simulink library "Pitch_System_Lib"  (Simulink 7.9)
settings: Solver=ode45  StartTime=0.0  StopTime=10.0  RelTol=1e-3
undefined symbols (not defined in the file or in its folder): WT_Params
libraries: mblibv1 x78, Pitch_Actuation_Lib x2, Pitch_System_Lib x1
(part 1 of 5)
Description:
  | Copyright 2011 MathWorks, Inc.
settings Model: Creator=smiller  LastModifiedBy=smiller

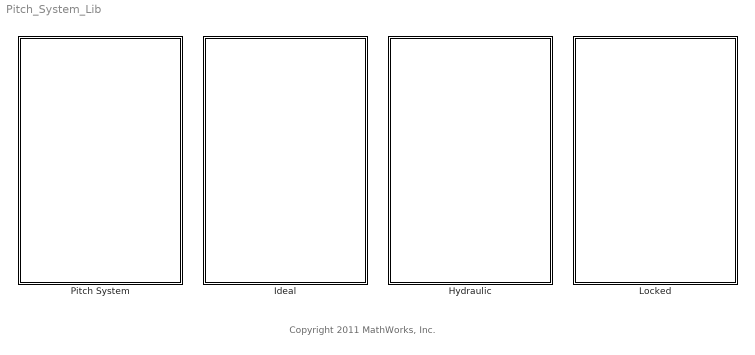
== system Pitch_System_Lib ==
  note: Copyright 2011 MathWorks, Inc.
  Hydraulic : Subsystem
      mask Display: image(imread('Pitch_Hydraulic_IMAGE.jpg'));
  Ideal : Subsystem
      mask Display: image(imread('Pitch_Ideal_IMAGE.jpg'));
  Locked : Subsystem
      mask Display: image(imread('Pitch_Locked_IMAGE.jpg'));
  Pitch System : Subsystem  BlockChoice=Hydraulic
      settings: TemplateBlock=self  MemberBlocks=Hydraulic,Ideal,Locked

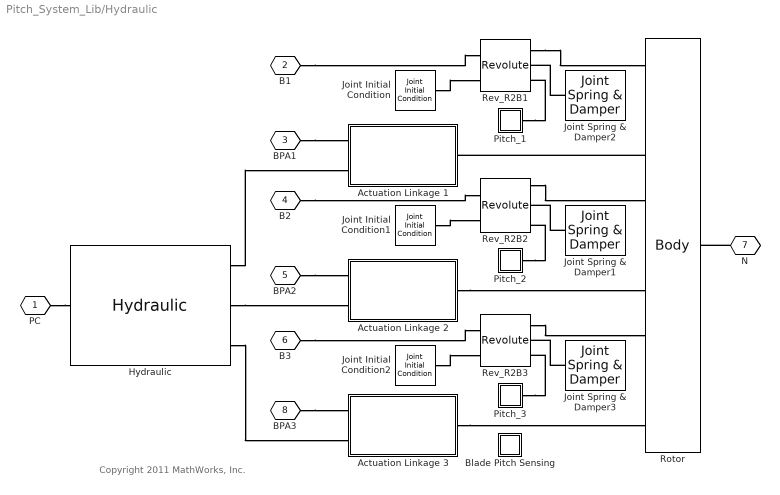
== system Pitch_System_Lib/Hydraulic ==
  note: Copyright 2011 MathWorks, Inc.
  Actuation Linkage 1 : Subsystem
      mask Display: image(imread('Pitch_Hydraulic_Linkage_IMAGE.jpg'));
  Actuation Linkage 2 : Subsystem
      mask Display: image(imread('Pitch_Hydraulic_Linkage_IMAGE.jpg'));
  Actuation Linkage 3 : Subsystem
      mask Display: image(imread('Pitch_Hydraulic_Linkage_IMAGE.jpg'));
  Blade Pitch Sensing : Subsystem
      mask Display: disp('S')
  Hydraulic : Pitch_Actuation_Lib/Hydraulic  SystemSampleTime=-1
  Joint Initial Condition : mblibv1/Sensors &  Actuators/Joint Initial Condition  SystemSampleTime=-1  UpdateFromCAD=off  LeftPortType=blob  RightPortType=blob  PhysicalDomain=mechanical  DialogClass=InitialConditionBlock  InitialConditions=P1$false$0$m$deg$0$m/s$deg/s#P2$false$0$m$deg$0$m/s$deg/s#P3$false$0$m$deg$0$m/s$deg/s#R1$true$0$m$deg$0$m/s$deg/s#R2$false$0$m$deg$0$m/s$deg/s#R3$false$0$m$deg$0$m/s$deg/s#S$false$0$m$deg$0$m/s$deg/s  P1PIC=0  P1VIC=0  P2PIC=0  P2VIC=0  P3PIC=0  P3VIC=0  R1PIC=0  R1VIC=0  R2PIC=0  R2VIC=0  R3PIC=0  R3VIC=0  SPIC=0  SVIC=0
  Joint Initial Condition1 : mblibv1/Sensors &  Actuators/Joint Initial Condition  SystemSampleTime=-1  UpdateFromCAD=off  LeftPortType=blob  RightPortType=blob  PhysicalDomain=mechanical  DialogClass=InitialConditionBlock  InitialConditions=P1$false$0$m$deg$0$m/s$deg/s#P2$false$0$m$deg$0$m/s$deg/s#P3$false$0$m$deg$0$m/s$deg/s#R1$true$0$m$deg$0$m/s$deg/s#R2$false$0$m$deg$0$m/s$deg/s#R3$false$0$m$deg$0$m/s$deg/s#S$false$0$m$deg$0$m/s$deg/s  P1PIC=0  P1VIC=0  P2PIC=0  P2VIC=0  P3PIC=0  P3VIC=0  R1PIC=0  R1VIC=0  R2PIC=0  R2VIC=0  R3PIC=0  R3VIC=0  SPIC=0  SVIC=0
  Joint Initial Condition2 : mblibv1/Sensors &  Actuators/Joint Initial Condition  SystemSampleTime=-1  UpdateFromCAD=off  LeftPortType=blob  RightPortType=blob  PhysicalDomain=mechanical  DialogClass=InitialConditionBlock  InitialConditions=P1$false$0$m$deg$0$m/s$deg/s#P2$false$0$m$deg$0$m/s$deg/s#P3$false$0$m$deg$0$m/s$deg/s#R1$true$0$m$deg$0$m/s$deg/s#R2$false$0$m$deg$0$m/s$deg/s#R3$false$0$m$deg$0$m/s$deg/s#S$false$0$m$deg$0$m/s$deg/s  P1PIC=0  P1VIC=0  P2PIC=0  P2VIC=0  P3PIC=0  P3VIC=0  R1PIC=0  R1VIC=0  R2PIC=0  R2VIC=0  R3PIC=0  R3VIC=0  SPIC=0  SVIC=0
  Joint Spring & Damper1 : mblibv1/Force  Elements/Joint Spring & Damper  SystemSampleTime=-1  UpdateFromCAD=off  DialogClass=JointSpringDamper  JFEParameters=P1$false$0$0$0$m$m/s$N$deg$deg/s$N*m#P2$false$0$0$0$m$m/s$N$deg$deg/s$N*m#P3$false$0$0$0$m$m/s$N$deg$deg/s$N*m#R1$true$0$WT_Params.Blade.damping$0$m$m/s$N$deg$deg/s$N*m#R2$false$0$0$0$m$m/s$N$deg$deg/s$N*m#R3$false$0$0$0$m$m/s$N$deg$deg/s$N*m#S$false$0$0$0$m$m/s$N$deg$deg/s$N*m
  Joint Spring & Damper2 : mblibv1/Force  Elements/Joint Spring & Damper  SystemSampleTime=-1  UpdateFromCAD=off  DialogClass=JointSpringDamper  JFEParameters=P1$false$0$0$0$m$m/s$N$deg$deg/s$N*m#P2$false$0$0$0$m$m/s$N$deg$deg/s$N*m#P3$false$0$0$0$m$m/s$N$deg$deg/s$N*m#R1$true$0$WT_Params.Blade.damping$0$m$m/s$N$deg$deg/s$N*m#R2$false$0$0$0$m$m/s$N$deg$deg/s$N*m#R3$false$0$0$0$m$m/s$N$deg$deg/s$N*m#S$false$0$0$0$m$m/s$N$deg$deg/s$N*m
  Joint Spring & Damper3 : mblibv1/Force  Elements/Joint Spring & Damper  SystemSampleTime=-1  UpdateFromCAD=off  DialogClass=JointSpringDamper  JFEParameters=P1$false$0$0$0$m$m/s$N$deg$deg/s$N*m#P2$false$0$0$0$m$m/s$N$deg$deg/s$N*m#P3$false$0$0$0$m$m/s$N$deg$deg/s$N*m#R1$true$0$WT_Params.Blade.damping$0$m$m/s$N$deg$deg/s$N*m#R2$false$0$0$0$m$m/s$N$deg$deg/s$N*m#R3$false$0$0$0$m$m/s$N$deg$deg/s$N*m#S$false$0$0$0$m$m/s$N$deg$deg/s$N*m
  Pitch_1 : Subsystem
  Pitch_2 : Subsystem
  Pitch_3 : Subsystem
  Rev_R2B1 : mblibv1/Joints/Revolute  LConnTagsString=__newl0|SA1|SA2  RConnTagsString=__newr0|SA1  UpdateFromCAD=off  NumSAPorts=3  CutJoint=off  MarkAsCut=off  Primitives=prismatic  PrimitiveProps=R1$Base$[0 -1 0]$revolute  DialogClass=JointBlock  R1Axis=[0 -1 0]
  Rev_R2B2 : mblibv1/Joints/Revolute  LConnTagsString=__newl0|SA1|SA2  RConnTagsString=__newr0|SA1  UpdateFromCAD=off  NumSAPorts=3  CutJoint=off  MarkAsCut=off  Primitives=prismatic  PrimitiveProps=R1$Base$[0 -1 0]$revolute  DialogClass=JointBlock  R1Axis=[0 -1 0]
  Rev_R2B3 : mblibv1/Joints/Revolute  LConnTagsString=__newl0|SA1|SA2  RConnTagsString=__newr0|SA1  UpdateFromCAD=off  NumSAPorts=3  CutJoint=off  MarkAsCut=off  Primitives=prismatic  PrimitiveProps=R1$Base$[0 -1 0]$revolute  DialogClass=JointBlock  R1Axis=[0 -1 0]
  Rotor : mblibv1/Bodies/Body  LConnTagsString=CS4|CS10|CS14|CS5|CS11|CS16|CS6|CS12|CS18  RConnTagsString=CG  UpdateFromCAD=off  DialogClass=MechanicalBodyBlock  Mass=WT_Params.Rotor.mass  MassUnits=kg  InertiaUnits=kg*m^2  Inertia=WT_Params.Rotor.inertia  Shape=Cylinder  ShapeDims=[1 1]  ShapeUnits=m  ShapeUse=false  Density=1  DensityUnits=kg/m^3  DensityUse=false  GraphicsMode=MACHINE_DEFAULT  BodyColorSelMode=COLORPALETTE  BodyColor=[1 1 1]  AttachedToCS=CG  CG=Right$CG$[0 0 0]$Adjoining$Adjoining$m$[0 0 0]$Euler X-Y-Z$deg$Adjoining$true$none  WorkingFrames=Right$CS19$[-WT_Params.Rotor.Geometry.length 0 0]$CG$CG$m$[0 0 0]$Euler X-Y-Z$deg$Adjoining$false$none#Left$CS1$[0 0 0]$CG$CG$m$[0 0 0]$Euler X-Y-Z$deg$CG$false$none#Left$CS4$[0 WT_Params.Rotor.radius 0]$CS1$CS1$m$[0 0 0]$Euler X-Y-Z$deg$CS1$true$none#Left$CS7$[0 0 0]$CG$CG$m$[60 0 0]$Euler X-Y-Z$deg$CG$false$none#Left$CS10$[0 WT_Params.Rotor.radius 0]$CS7$CS7$m$[0 0 0]$Euler X-Y-Z$deg$CS7$true$none#Left$CS13$[-WT_Params.Rotor.Pitch_Actuator_Offset.x 0 WT_Params.Rotor.Pitch_Actuator_Offset.z]$CG$CG$m$[WT_Params.Rotor.Pitch_Actuator_Offset.angle 0 0]$Euler X-Y-Z$deg$CG$false$none#Left$CS14$[0 WT_Params.Rotor.Pitch_Actuator_Offset.y 0]$CS13$CS13$m$[0 0 0]$Euler X-Y-Z$deg$CS13$true$none#Left$CS2$[0 0 0]$CG$CG$m$[120 0 0]$Euler X-Y-Z$deg$CG$false$none#Left$CS5$[0 WT_Params.Rotor.radius 0]$CS2$CS2$m$[0 0 0]$Euler X-Y-Z$deg$CS2$true$none#Left$CS8$[0 0 0]$CG$CG$m$[180 0 0]$Euler X-Y-Z$deg$CG$false$none#Left$CS11$[0 WT_Params.Rotor.radius 0]$CS8$CS8$m$[0 0 0]$Euler X-Y-Z$deg$CS8$true$none#Left$CS15$[-WT_Params.Rotor.Pitch_Actuator_Offset.x 0 0]$CG$CG$m$[WT_Params.Rotor.Pitch_Actuator_Offset.angle+120 0 0]$Euler X-Y-Z$deg$CG$false$none#Left$CS16$[0 WT_Params.Rotor.Pitch_Actuator_Offset.y WT_Params.Rotor.Pitch_Actuator_Offset.z]$CS15$CS15$m$[0 0 0]$Euler X-Y-Z$deg$CS15$true$none#Left$CS3$[0 0 0]$CG$CG$m$[240 0 0]$Euler X-Y-Z$deg$CG$false$none#Left$CS6$[0 WT_Params.Rotor.radius 0]$CS3$CS3$m$[0 0 0]$Euler X-Y-Z$deg$CS3$true$none#Left$CS9$[0 0 0]$CG$CG$m$[300 0 0]$Euler X-Y-Z$deg$CG$false$none#Left$CS12$[0 WT_Params.Rotor.radius 0]$CS9$CS9$m$[0 0 0]$Euler X-Y-Z$deg$CS9$true$none#Left$CS17$[-WT_Params.Rotor.Pitch_Actuator_Offset.x 0 0]$CG$CG$m$[WT_Params.Rotor.Pitch_Actuator_Offset.angle+240 0 0]$Euler X-Y-Z$deg$CG$false$none#Left$CS18$[0 WT_Params.Rotor.Pitch_Actuator_Offset.y WT_Params.Rotor.Pitch_Actuator_Offset.z]$CS17$CS17$m$[0 0 0]$Euler X-Y-Z$deg$CS17$true$none  CGPos=[0 0 0]  CGRot=[0 0 0]  CS0Pos=[]  CS0Rot=[]  CS1Pos=[0 0 0]  CS1Rot=[0 0 0]  CS2Pos=[0 0 0]  CS2Rot=[120 0 0]  CS3Pos=[0 0 0]  CS3Rot=[240 0 0]  CS4Pos=[0 WT_Params.Rotor.radius 0]  CS4Rot=[0 0 0]  CS5Pos=[0 WT_Params.Rotor.radius 0]  CS5Rot=[0 0 0]  CS6Pos=[0 WT_Params.Rotor.radius 0]  CS6Rot=[0 0 0]  CS7Pos=[0 0 0]  CS7Rot=[60 0 0]  CS8Pos=[0 0 0]  CS8Rot=[180 0 0]  CS9Pos=[0 0 0]  CS9Rot=[300 0 0]  CS10Pos=[0 WT_Params.Rotor.radius 0]  CS10Rot=[0 0 0]  CS11Pos=[0 WT_Params.Rotor.radius 0]  CS11Rot=[0 0 0]  CS12Pos=[0 WT_Params.Rotor.radius 0]  CS12Rot=[0 0 0]  CS13Pos=[-WT_Params.Rotor.Pitch_Actuator_Offset.x 0 WT_Params.Rotor.Pitch_Actuator_Offset.z]  CS13Rot=[WT_Params.Rotor.Pitch_Actuator_Offset.angle 0 0]  CS14Pos=[0 WT_Params.Rotor.Pitch_Actuator_Offset.y 0]  CS14Rot=[0 0 0]  CS15Pos=[-WT_Params.Rotor.Pitch_Actuator_Offset.x 0 0]  CS15Rot=[WT_Params.Rotor.Pitch_Actuator_Offset.angle+120 0 0]  CS16Pos=[0 WT_Params.Rotor.Pitch_Actuator_Offset.y WT_Params.Rotor.Pitch_Actuator_Offset.z]  CS16Rot=[0 0 0]  CS17Pos=[-WT_Params.Rotor.Pitch_Actuator_Offset.x 0 0]  CS17Rot=[WT_Params.Rotor.Pitch_Actuator_Offset.angle+240 0 0]  CS18Pos=[0 WT_Params.Rotor.Pitch_Actuator_Offset.y WT_Params.Rotor.Pitch_Actuator_Offset.z]  CS18Rot=[0 0 0]  CS19Pos=[-WT_Params.Rotor.Geometry.length 0 0]  CS19Rot=[0 0 0]  CS20Pos=[]  CS20Rot=[]
  PC : PMIOPort  Tag=PMCPort  Port=1  Side=Left
  B1 : PMIOPort  Tag=PMCPort  Port=2  Side=Left
  BPA1 : PMIOPort  Tag=PMCPort  Port=3  Side=Left
  B2 : PMIOPort  Tag=PMCPort  Port=4  Side=Left
  BPA2 : PMIOPort  Tag=PMCPort  Port=5  Side=Left
  B3 : PMIOPort  Tag=PMCPort  Port=6  Side=Left
  N : PMIOPort  Tag=PMCPort  Port=7  Side=Right
  BPA3 : PMIOPort  Tag=PMCPort  Port=8  Side=Left
  connections:
  Pitch_1/LConn1 -- Rev_R2B1/LConn3
  B3/RConn1 -- Rev_R2B3/RConn1
  B2/RConn1 -- Rev_R2B2/RConn1
  B1/RConn1 -- Rev_R2B1/RConn1
  Rev_R2B1/LConn1 -- Rotor/LConn1
  Rev_R2B2/LConn1 -- Rotor/LConn4
  Rev_R2B3/LConn1 -- Rotor/LConn7
  Rotor/LConn3 -- Actuation Linkage 1/RConn1
  Hydraulic/RConn1 -- Actuation Linkage 1/LConn2
  BPA2/RConn1 -- Actuation Linkage 2/LConn1
  Actuation Linkage 3/RConn1 -- Rotor/LConn9
  BPA3/RConn1 -- Actuation Linkage 3/LConn1
  Actuation Linkage 2/RConn1 -- Rotor/LConn6
  BPA1/RConn1 -- Actuation Linkage 1/LConn1
  Hydraulic/RConn3 -- Actuation Linkage 3/LConn2
  PC/RConn1 -- Hydraulic/LConn1
  Hydraulic/RConn2 -- Actuation Linkage 2/LConn2
  Joint Spring & Damper1/LConn1 -- Rev_R2B2/LConn2
  Joint Spring & Damper3/LConn1 -- Rev_R2B3/LConn2
  Joint Spring & Damper2/LConn1 -- Rev_R2B1/LConn2
  Joint Initial Condition/RConn1 -- Rev_R2B1/RConn2
  Joint Initial Condition1/RConn1 -- Rev_R2B2/RConn2
  Joint Initial Condition2/RConn1 -- Rev_R2B3/RConn2
  Pitch_2/LConn1 -- Rev_R2B2/LConn3
  Pitch_3/LConn1 -- Rev_R2B3/LConn3
  N/RConn1 -- Rotor/RConn1

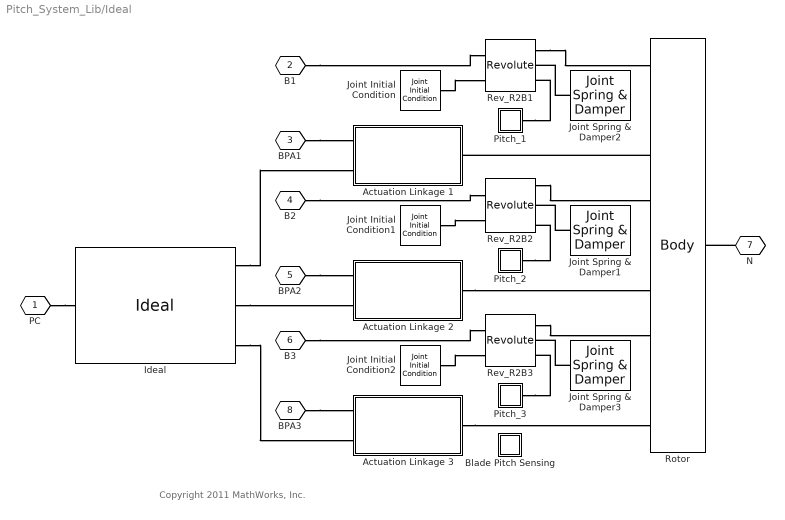
== system Pitch_System_Lib/Ideal ==
  note: Copyright 2011 MathWorks, Inc.
  Actuation Linkage 1 : Subsystem
      mask Display: image(imread('Pitch_Ideal_Linkage_IMAGE.jpg'));
  Actuation Linkage 2 : Subsystem
      mask Display: image(imread('Pitch_Ideal_Linkage_IMAGE.jpg'));
  Actuation Linkage 3 : Subsystem
      mask Display: image(imread('Pitch_Ideal_Linkage_IMAGE.jpg'));
  Blade Pitch Sensing : Subsystem
      mask Display: disp('S')
  Ideal : Pitch_Actuation_Lib/Ideal  SystemSampleTime=-1
  Joint Initial Condition : mblibv1/Sensors &  Actuators/Joint Initial Condition  SystemSampleTime=-1  UpdateFromCAD=off  LeftPortType=blob  RightPortType=blob  PhysicalDomain=mechanical  DialogClass=InitialConditionBlock  InitialConditions=P1$false$0$m$deg$0$m/s$deg/s#P2$false$0$m$deg$0$m/s$deg/s#P3$false$0$m$deg$0$m/s$deg/s#R1$true$0$m$deg$0$m/s$deg/s#R2$false$0$m$deg$0$m/s$deg/s#R3$false$0$m$deg$0$m/s$deg/s#S$false$0$m$deg$0$m/s$deg/s  P1PIC=0  P1VIC=0  P2PIC=0  P2VIC=0  P3PIC=0  P3VIC=0  R1PIC=0  R1VIC=0  R2PIC=0  R2VIC=0  R3PIC=0  R3VIC=0  SPIC=0  SVIC=0
  Joint Initial Condition1 : mblibv1/Sensors &  Actuators/Joint Initial Condition  SystemSampleTime=-1  UpdateFromCAD=off  LeftPortType=blob  RightPortType=blob  PhysicalDomain=mechanical  DialogClass=InitialConditionBlock  InitialConditions=P1$false$0$m$deg$0$m/s$deg/s#P2$false$0$m$deg$0$m/s$deg/s#P3$false$0$m$deg$0$m/s$deg/s#R1$true$0$m$deg$0$m/s$deg/s#R2$false$0$m$deg$0$m/s$deg/s#R3$false$0$m$deg$0$m/s$deg/s#S$false$0$m$deg$0$m/s$deg/s  P1PIC=0  P1VIC=0  P2PIC=0  P2VIC=0  P3PIC=0  P3VIC=0  R1PIC=0  R1VIC=0  R2PIC=0  R2VIC=0  R3PIC=0  R3VIC=0  SPIC=0  SVIC=0
  Joint Initial Condition2 : mblibv1/Sensors &  Actuators/Joint Initial Condition  SystemSampleTime=-1  UpdateFromCAD=off  LeftPortType=blob  RightPortType=blob  PhysicalDomain=mechanical  DialogClass=InitialConditionBlock  InitialConditions=P1$false$0$m$deg$0$m/s$deg/s#P2$false$0$m$deg$0$m/s$deg/s#P3$false$0$m$deg$0$m/s$deg/s#R1$true$0$m$deg$0$m/s$deg/s#R2$false$0$m$deg$0$m/s$deg/s#R3$false$0$m$deg$0$m/s$deg/s#S$false$0$m$deg$0$m/s$deg/s  P1PIC=0  P1VIC=0  P2PIC=0  P2VIC=0  P3PIC=0  P3VIC=0  R1PIC=0  R1VIC=0  R2PIC=0  R2VIC=0  R3PIC=0  R3VIC=0  SPIC=0  SVIC=0
  Joint Spring & Damper1 : mblibv1/Force  Elements/Joint Spring & Damper  SystemSampleTime=-1  UpdateFromCAD=off  DialogClass=JointSpringDamper  JFEParameters=P1$false$0$0$0$m$m/s$N$deg$deg/s$N*m#P2$false$0$0$0$m$m/s$N$deg$deg/s$N*m#P3$false$0$0$0$m$m/s$N$deg$deg/s$N*m#R1$true$0$WT_Params.Blade.damping$0$m$m/s$N$deg$deg/s$N*m#R2$false$0$0$0$m$m/s$N$deg$deg/s$N*m#R3$false$0$0$0$m$m/s$N$deg$deg/s$N*m#S$false$0$0$0$m$m/s$N$deg$deg/s$N*m
  Joint Spring & Damper2 : mblibv1/Force  Elements/Joint Spring & Damper  SystemSampleTime=-1  UpdateFromCAD=off  DialogClass=JointSpringDamper  JFEParameters=P1$false$0$0$0$m$m/s$N$deg$deg/s$N*m#P2$false$0$0$0$m$m/s$N$deg$deg/s$N*m#P3$false$0$0$0$m$m/s$N$deg$deg/s$N*m#R1$true$0$WT_Params.Blade.damping$0$m$m/s$N$deg$deg/s$N*m#R2$false$0$0$0$m$m/s$N$deg$deg/s$N*m#R3$false$0$0$0$m$m/s$N$deg$deg/s$N*m#S$false$0$0$0$m$m/s$N$deg$deg/s$N*m
  Joint Spring & Damper3 : mblibv1/Force  Elements/Joint Spring & Damper  SystemSampleTime=-1  UpdateFromCAD=off  DialogClass=JointSpringDamper  JFEParameters=P1$false$0$0$0$m$m/s$N$deg$deg/s$N*m#P2$false$0$0$0$m$m/s$N$deg$deg/s$N*m#P3$false$0$0$0$m$m/s$N$deg$deg/s$N*m#R1$true$0$WT_Params.Blade.damping$0$m$m/s$N$deg$deg/s$N*m#R2$false$0$0$0$m$m/s$N$deg$deg/s$N*m#R3$false$0$0$0$m$m/s$N$deg$deg/s$N*m#S$false$0$0$0$m$m/s$N$deg$deg/s$N*m
  Pitch_1 : Subsystem
  Pitch_2 : Subsystem
  Pitch_3 : Subsystem
  Rev_R2B1 : mblibv1/Joints/Revolute  LConnTagsString=__newl0|SA1|SA2  RConnTagsString=__newr0|SA1  UpdateFromCAD=off  NumSAPorts=3  CutJoint=off  MarkAsCut=off  Primitives=prismatic  PrimitiveProps=R1$Base$[0 -1 0]$revolute  DialogClass=JointBlock  R1Axis=[0 -1 0]
  Rev_R2B2 : mblibv1/Joints/Revolute  LConnTagsString=__newl0|SA1|SA2  RConnTagsString=__newr0|SA1  UpdateFromCAD=off  NumSAPorts=3  CutJoint=off  MarkAsCut=off  Primitives=prismatic  PrimitiveProps=R1$Base$[0 -1 0]$revolute  DialogClass=JointBlock  R1Axis=[0 -1 0]
  Rev_R2B3 : mblibv1/Joints/Revolute  LConnTagsString=__newl0|SA1|SA2  RConnTagsString=__newr0|SA1  UpdateFromCAD=off  NumSAPorts=3  CutJoint=off  MarkAsCut=off  Primitives=prismatic  PrimitiveProps=R1$Base$[0 -1 0]$revolute  DialogClass=JointBlock  R1Axis=[0 -1 0]
  Rotor : mblibv1/Bodies/Body  LConnTagsString=CS4|CS10|CS14|CS5|CS11|CS16|CS6|CS12|CS18  RConnTagsString=CG  UpdateFromCAD=off  DialogClass=MechanicalBodyBlock  Mass=WT_Params.Rotor.mass  MassUnits=kg  InertiaUnits=kg*m^2  Inertia=WT_Params.Rotor.inertia  Shape=Cylinder  ShapeDims=[1 1]  ShapeUnits=m  ShapeUse=false  Density=1  DensityUnits=kg/m^3  DensityUse=false  GraphicsMode=MACHINE_DEFAULT  BodyColorSelMode=COLORPALETTE  BodyColor=[1 1 1]  AttachedToCS=CG  CG=Right$CG$[0 0 0]$Adjoining$Adjoining$m$[0 0 0]$Euler X-Y-Z$deg$Adjoining$true$none  WorkingFrames=Right$CS19$[-WT_Params.Rotor.Geometry.length 0 0]$CG$CG$m$[0 0 0]$Euler X-Y-Z$deg$Adjoining$false$none#Left$CS1$[0 0 0]$CG$CG$m$[0 0 0]$Euler X-Y-Z$deg$CG$false$none#Left$CS4$[0 WT_Params.Rotor.radius 0]$CS1$CS1$m$[0 0 0]$Euler X-Y-Z$deg$CS1$true$none#Left$CS7$[0 0 0]$CG$CG$m$[60 0 0]$Euler X-Y-Z$deg$CG$false$none#Left$CS10$[0 WT_Params.Rotor.radius 0]$CS7$CS7$m$[0 0 0]$Euler X-Y-Z$deg$CS7$true$none#Left$CS13$[-WT_Params.Rotor.Pitch_Actuator_Offset.x 0 WT_Params.Rotor.Pitch_Actuator_Offset.z]$CG$CG$m$[WT_Params.Rotor.Pitch_Actuator_Offset.angle 0 0]$Euler X-Y-Z$deg$CG$false$none#Left$CS14$[0 WT_Params.Rotor.Pitch_Actuator_Offset.y 0]$CS13$CS13$m$[0 0 0]$Euler X-Y-Z$deg$CS13$true$none#Left$CS2$[0 0 0]$CG$CG$m$[120 0 0]$Euler X-Y-Z$deg$CG$false$none#Left$CS5$[0 WT_Params.Rotor.radius 0]$CS2$CS2$m$[0 0 0]$Euler X-Y-Z$deg$CS2$true$none#Left$CS8$[0 0 0]$CG$CG$m$[180 0 0]$Euler X-Y-Z$deg$CG$false$none#Left$CS11$[0 WT_Params.Rotor.radius 0]$CS8$CS8$m$[0 0 0]$Euler X-Y-Z$deg$CS8$true$none#Left$CS15$[-WT_Params.Rotor.Pitch_Actuator_Offset.x 0 0]$CG$CG$m$[WT_Params.Rotor.Pitch_Actuator_Offset.angle+120 0 0]$Euler X-Y-Z$deg$CG$false$none#Left$CS16$[0 WT_Params.Rotor.Pitch_Actuator_Offset.y WT_Params.Rotor.Pitch_Actuator_Offset.z]$CS15$CS15$m$[0 0 0]$Euler X-Y-Z$deg$CS15$true$none#Left$CS3$[0 0 0]$CG$CG$m$[240 0 0]$Euler X-Y-Z$deg$CG$false$none#Left$CS6$[0 WT_Params.Rotor.radius 0]$CS3$CS3$m$[0 0 0]$Euler X-Y-Z$deg$CS3$true$none#Left$CS9$[0 0 0]$CG$CG$m$[300 0 0]$Euler X-Y-Z$deg$CG$false$none#Left$CS12$[0 WT_Params.Rotor.radius 0]$CS9$CS9$m$[0 0 0]$Euler X-Y-Z$deg$CS9$true$none#Left$CS17$[-WT_Params.Rotor.Pitch_Actuator_Offset.x 0 0]$CG$CG$m$[WT_Params.Rotor.Pitch_Actuator_Offset.angle+240 0 0]$Euler X-Y-Z$deg$CG$false$none#Left$CS18$[0 WT_Params.Rotor.Pitch_Actuator_Offset.y WT_Params.Rotor.Pitch_Actuator_Offset.z]$CS17$CS17$m$[0 0 0]$Euler X-Y-Z$deg$CS17$true$none  CGPos=[0 0 0]  CGRot=[0 0 0]  CS0Pos=[]  CS0Rot=[]  CS1Pos=[0 0 0]  CS1Rot=[0 0 0]  CS2Pos=[0 0 0]  CS2Rot=[120 0 0]  CS3Pos=[0 0 0]  CS3Rot=[240 0 0]  CS4Pos=[0 WT_Params.Rotor.radius 0]  CS4Rot=[0 0 0]  CS5Pos=[0 WT_Params.Rotor.radius 0]  CS5Rot=[0 0 0]  CS6Pos=[0 WT_Params.Rotor.radius 0]  CS6Rot=[0 0 0]  CS7Pos=[0 0 0]  CS7Rot=[60 0 0]  CS8Pos=[0 0 0]  CS8Rot=[180 0 0]  CS9Pos=[0 0 0]  CS9Rot=[300 0 0]  CS10Pos=[0 WT_Params.Rotor.radius 0]  CS10Rot=[0 0 0]  CS11Pos=[0 WT_Params.Rotor.radius 0]  CS11Rot=[0 0 0]  CS12Pos=[0 WT_Params.Rotor.radius 0]  CS12Rot=[0 0 0]  CS13Pos=[-WT_Params.Rotor.Pitch_Actuator_Offset.x 0 WT_Params.Rotor.Pitch_Actuator_Offset.z]  CS13Rot=[WT_Params.Rotor.Pitch_Actuator_Offset.angle 0 0]  CS14Pos=[0 WT_Params.Rotor.Pitch_Actuator_Offset.y 0]  CS14Rot=[0 0 0]  CS15Pos=[-WT_Params.Rotor.Pitch_Actuator_Offset.x 0 0]  CS15Rot=[WT_Params.Rotor.Pitch_Actuator_Offset.angle+120 0 0]  CS16Pos=[0 WT_Params.Rotor.Pitch_Actuator_Offset.y WT_Params.Rotor.Pitch_Actuator_Offset.z]  CS16Rot=[0 0 0]  CS17Pos=[-WT_Params.Rotor.Pitch_Actuator_Offset.x 0 0]  CS17Rot=[WT_Params.Rotor.Pitch_Actuator_Offset.angle+240 0 0]  CS18Pos=[0 WT_Params.Rotor.Pitch_Actuator_Offset.y WT_Params.Rotor.Pitch_Actuator_Offset.z]  CS18Rot=[0 0 0]  CS19Pos=[-WT_Params.Rotor.Geometry.length 0 0]  CS19Rot=[0 0 0]  CS20Pos=[]  CS20Rot=[]
  PC : PMIOPort  Tag=PMCPort  Port=1  Side=Left
  B1 : PMIOPort  Tag=PMCPort  Port=2  Side=Left
  BPA1 : PMIOPort  Tag=PMCPort  Port=3  Side=Left
  B2 : PMIOPort  Tag=PMCPort  Port=4  Side=Left
  BPA2 : PMIOPort  Tag=PMCPort  Port=5  Side=Left
  B3 : PMIOPort  Tag=PMCPort  Port=6  Side=Left
  N : PMIOPort  Tag=PMCPort  Port=7  Side=Right
  BPA3 : PMIOPort  Tag=PMCPort  Port=8  Side=Left
  connections:
  N/RConn1 -- Rotor/RConn1
  Pitch_3/LConn1 -- Rev_R2B3/LConn3
  Pitch_2/LConn1 -- Rev_R2B2/LConn3
  Joint Initial Condition2/RConn1 -- Rev_R2B3/RConn2
  Joint Initial Condition1/RConn1 -- Rev_R2B2/RConn2
  Joint Initial Condition/RConn1 -- Rev_R2B1/RConn2
  Joint Spring & Damper2/LConn1 -- Rev_R2B1/LConn2
  Joint Spring & Damper3/LConn1 -- Rev_R2B3/LConn2
  Joint Spring & Damper1/LConn1 -- Rev_R2B2/LConn2
  Ideal/RConn2 -- Actuation Linkage 2/LConn2
  PC/RConn1 -- Ideal/LConn1
  Ideal/RConn3 -- Actuation Linkage 3/LConn2
  BPA1/RConn1 -- Actuation Linkage 1/LConn1
  Actuation Linkage 2/RConn1 -- Rotor/LConn6
  BPA3/RConn1 -- Actuation Linkage 3/LConn1
  Actuation Linkage 3/RConn1 -- Rotor/LConn9
  BPA2/RConn1 -- Actuation Linkage 2/LConn1
  Ideal/RConn1 -- Actuation Linkage 1/LConn2
  Rotor/LConn3 -- Actuation Linkage 1/RConn1
  Rev_R2B3/LConn1 -- Rotor/LConn7
  Rev_R2B2/LConn1 -- Rotor/LConn4
  Rev_R2B1/LConn1 -- Rotor/LConn1
  B1/RConn1 -- Rev_R2B1/RConn1
  B2/RConn1 -- Rev_R2B2/RConn1
  B3/RConn1 -- Rev_R2B3/RConn1
  Pitch_1/LConn1 -- Rev_R2B1/LConn3

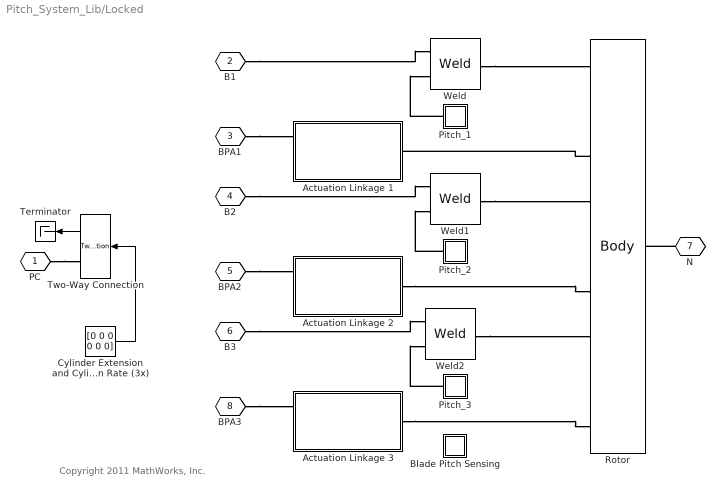
== system Pitch_System_Lib/Locked ==
  note: Copyright 2011 MathWorks, Inc.
  Actuation Linkage 1 : Subsystem
      mask Display: image(imread('Pitch_Locked_Linkage_IMAGE.jpg'))
  Actuation Linkage 2 : Subsystem
      mask Display: image(imread('Pitch_Locked_Linkage_IMAGE.jpg'))
  Actuation Linkage 3 : Subsystem
      mask Display: image(imread('Pitch_Locked_Linkage_IMAGE.jpg'))
  Blade Pitch Sensing : Subsystem
      mask Display: disp('S')
  Cylinder Extension and Cylinder Extension Rate (3x) : Constant  Value=[0 0 0 0 0 0]
  Pitch_1 : Subsystem
  Pitch_2 : Subsystem
  Pitch_3 : Subsystem
  Rotor : mblibv1/Bodies/Body  LConnTagsString=CS4|CS10|CS14|CS5|CS11|CS16|CS6|CS12|CS18  RConnTagsString=CG  UpdateFromCAD=off  DialogClass=MechanicalBodyBlock  Mass=WT_Params.Rotor.mass  MassUnits=kg  InertiaUnits=kg*m^2  Inertia=WT_Params.Rotor.inertia  Shape=Cylinder  ShapeDims=[1 1]  ShapeUnits=m  ShapeUse=false  Density=1  DensityUnits=kg/m^3  DensityUse=false  GraphicsMode=MACHINE_DEFAULT  BodyColorSelMode=COLORPALETTE  BodyColor=[1 1 1]  AttachedToCS=CG  CG=Right$CG$[0 0 0]$Adjoining$Adjoining$m$[0 0 0]$Euler X-Y-Z$deg$Adjoining$true$none  WorkingFrames=Right$CS19$[-WT_Params.Rotor.Geometry.length 0 0]$CG$CG$m$[0 0 0]$Euler X-Y-Z$deg$Adjoining$false$none#Left$CS1$[0 0 0]$CG$CG$m$[0 0 0]$Euler X-Y-Z$deg$CG$false$none#Left$CS4$[0 WT_Params.Rotor.radius 0]$CS1$CS1$m$[0 0 0]$Euler X-Y-Z$deg$CS1$true$none#Left$CS7$[0 0 0]$CG$CG$m$[60 0 0]$Euler X-Y-Z$deg$CG$false$none#Left$CS10$[0 WT_Params.Rotor.radius 0]$CS7$CS7$m$[0 0 0]$Euler X-Y-Z$deg$CS7$true$none#Left$CS13$[-WT_Params.Rotor.Pitch_Actuator_Offset.x 0 WT_Params.Rotor.Pitch_Actuator_Offset.z]$CG$CG$m$[WT_Params.Rotor.Pitch_Actuator_Offset.angle 0 0]$Euler X-Y-Z$deg$CG$false$none#Left$CS14$[0 WT_Params.Rotor.Pitch_Actuator_Offset.y 0]$CS13$CS13$m$[0 0 0]$Euler X-Y-Z$deg$CS13$true$none#Left$CS2$[0 0 0]$CG$CG$m$[120 0 0]$Euler X-Y-Z$deg$CG$false$none#Left$CS5$[0 WT_Params.Rotor.radius 0]$CS2$CS2$m$[0 0 0]$Euler X-Y-Z$deg$CS2$true$none#Left$CS8$[0 0 0]$CG$CG$m$[180 0 0]$Euler X-Y-Z$deg$CG$false$none#Left$CS11$[0 WT_Params.Rotor.radius 0]$CS8$CS8$m$[0 0 0]$Euler X-Y-Z$deg$CS8$true$none#Left$CS15$[-WT_Params.Rotor.Pitch_Actuator_Offset.x 0 0]$CG$CG$m$[WT_Params.Rotor.Pitch_Actuator_Offset.angle+120 0 0]$Euler X-Y-Z$deg$CG$false$none#Left$CS16$[0 WT_Params.Rotor.Pitch_Actuator_Offset.y WT_Params.Rotor.Pitch_Actuator_Offset.z]$CS15$CS15$m$[0 0 0]$Euler X-Y-Z$deg$CS15$true$none#Left$CS3$[0 0 0]$CG$CG$m$[240 0 0]$Euler X-Y-Z$deg$CG$false$none#Left$CS6$[0 WT_Params.Rotor.radius 0]$CS3$CS3$m$[0 0 0]$Euler X-Y-Z$deg$CS3$true$none#Left$CS9$[0 0 0]$CG$CG$m$[300 0 0]$Euler X-Y-Z$deg$CG$false$none#Left$CS12$[0 WT_Params.Rotor.radius 0]$CS9$CS9$m$[0 0 0]$Euler X-Y-Z$deg$CS9$true$none#Left$CS17$[-WT_Params.Rotor.Pitch_Actuator_Offset.x 0 0]$CG$CG$m$[WT_Params.Rotor.Pitch_Actuator_Offset.angle+240 0 0]$Euler X-Y-Z$deg$CG$false$none#Left$CS18$[0 WT_Params.Rotor.Pitch_Actuator_Offset.y WT_Params.Rotor.Pitch_Actuator_Offset.z]$CS17$CS17$m$[0 0 0]$Euler X-Y-Z$deg$CS17$true$none  CGPos=[0 0 0]  CGRot=[0 0 0]  CS0Pos=[]  CS0Rot=[]  CS1Pos=[0 0 0]  CS1Rot=[0 0 0]  CS2Pos=[0 0 0]  CS2Rot=[120 0 0]  CS3Pos=[0 0 0]  CS3Rot=[240 0 0]  CS4Pos=[0 WT_Params.Rotor.radius 0]  CS4Rot=[0 0 0]  CS5Pos=[0 WT_Params.Rotor.radius 0]  CS5Rot=[0 0 0]  CS6Pos=[0 WT_Params.Rotor.radius 0]  CS6Rot=[0 0 0]  CS7Pos=[0 0 0]  CS7Rot=[60 0 0]  CS8Pos=[0 0 0]  CS8Rot=[180 0 0]  CS9Pos=[0 0 0]  CS9Rot=[300 0 0]  CS10Pos=[0 WT_Params.Rotor.radius 0]  CS10Rot=[0 0 0]  CS11Pos=[0 WT_Params.Rotor.radius 0]  CS11Rot=[0 0 0]  CS12Pos=[0 WT_Params.Rotor.radius 0]  CS12Rot=[0 0 0]  CS13Pos=[-WT_Params.Rotor.Pitch_Actuator_Offset.x 0 WT_Params.Rotor.Pitch_Actuator_Offset.z]  CS13Rot=[WT_Params.Rotor.Pitch_Actuator_Offset.angle 0 0]  CS14Pos=[0 WT_Params.Rotor.Pitch_Actuator_Offset.y 0]  CS14Rot=[0 0 0]  CS15Pos=[-WT_Params.Rotor.Pitch_Actuator_Offset.x 0 0]  CS15Rot=[WT_Params.Rotor.Pitch_Actuator_Offset.angle+120 0 0]  CS16Pos=[0 WT_Params.Rotor.Pitch_Actuator_Offset.y WT_Params.Rotor.Pitch_Actuator_Offset.z]  CS16Rot=[0 0 0]  CS17Pos=[-WT_Params.Rotor.Pitch_Actuator_Offset.x 0 0]  CS17Rot=[WT_Params.Rotor.Pitch_Actuator_Offset.angle+240 0 0]  CS18Pos=[0 WT_Params.Rotor.Pitch_Actuator_Offset.y WT_Params.Rotor.Pitch_Actuator_Offset.z]  CS18Rot=[0 0 0]  CS19Pos=[-WT_Params.Rotor.Geometry.length 0 0]  CS19Rot=[0 0 0]  CS20Pos=[]  CS20Rot=[]
  Terminator : Terminator
  Two-Way Connection : TwoWayConnection
  Weld : mblibv1/Joints/Weld  LConnTagsString=__newl0|SA1  RConnTagsString=__newr0  UpdateFromCAD=off  NumSAPorts=1  CutJoint=off  MarkAsCut=off  Primitives=weld  PrimitiveProps=W$World$[0 0 0]$weld  DialogClass=JointBlock  WAxis=[0 0 0]
  Weld1 : mblibv1/Joints/Weld  LConnTagsString=__newl0|SA1  RConnTagsString=__newr0  UpdateFromCAD=off  NumSAPorts=1  CutJoint=off  MarkAsCut=off  Primitives=weld  PrimitiveProps=W$World$[0 0 0]$weld  DialogClass=JointBlock  WAxis=[0 0 0]
  Weld2 : mblibv1/Joints/Weld  LConnTagsString=__newl0|SA1  RConnTagsString=__newr0  UpdateFromCAD=off  NumSAPorts=1  CutJoint=off  MarkAsCut=off  Primitives=weld  PrimitiveProps=W$World$[0 0 0]$weld  DialogClass=JointBlock  WAxis=[0 0 0]
  PC : PMIOPort  Tag=PMCPort  Port=1  Side=Left
  B1 : PMIOPort  Tag=PMCPort  Port=2  Side=Left
  BPA1 : PMIOPort  Tag=PMCPort  Port=3  Side=Left
  B2 : PMIOPort  Tag=PMCPort  Port=4  Side=Left
  BPA2 : PMIOPort  Tag=PMCPort  Port=5  Side=Left
  B3 : PMIOPort  Tag=PMCPort  Port=6  Side=Left
  N : PMIOPort  Tag=PMCPort  Port=7  Side=Right
  BPA3 : PMIOPort  Tag=PMCPort  Port=8  Side=Left
  wires:
  Cylinder Extension and Cylinder Extension Rate (3x)/1 -> Two-Way Connection/1
  Two-Way Connection/1 -> Terminator/1
  connections:
  N/RConn1 -- Rotor/RConn1
  PC/RConn1 -- Two-Way Connection/RConn1
  BPA1/RConn1 -- Actuation Linkage 1/LConn1
  Actuation Linkage 2/RConn1 -- Rotor/LConn6
  BPA3/RConn1 -- Actuation Linkage 3/LConn1
  Actuation Linkage 3/RConn1 -- Rotor/LConn9
  BPA2/RConn1 -- Actuation Linkage 2/LConn1
  Rotor/LConn3 -- Actuation Linkage 1/RConn1
  Weld2/RConn1 -- Rotor/LConn7
  Weld1/RConn1 -- Rotor/LConn4
  Weld/RConn1 -- Rotor/LConn1
  B1/RConn1 -- Weld/LConn1
  B2/RConn1 -- Weld1/LConn1
  B3/RConn1 -- Weld2/LConn1
  Pitch_1/LConn1 -- Weld/LConn2
  Pitch_2/LConn1 -- Weld1/LConn2
  Pitch_3/LConn1 -- Weld2/LConn2

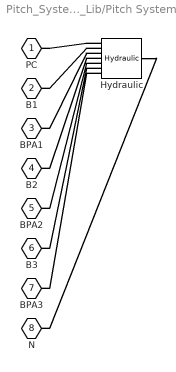
== system Pitch_System_Lib/Pitch System ==
  Hydraulic : Pitch_System_Lib/Hydraulic  SystemSampleTime=-1
  PC : PMIOPort  Port=1  Side=Left
  B1 : PMIOPort  Port=2  Side=Left
  BPA1 : PMIOPort  Port=3  Side=Left
  B2 : PMIOPort  Port=4  Side=Left
  BPA2 : PMIOPort  Port=5  Side=Left
  B3 : PMIOPort  Port=6  Side=Left
  BPA3 : PMIOPort  Port=7  Side=Left
  N : PMIOPort  Port=8  Side=Right
  connections:
  Hydraulic/LConn1 -- PC/RConn1
  Hydraulic/LConn2 -- B1/RConn1
  Hydraulic/LConn3 -- BPA1/RConn1
  Hydraulic/LConn4 -- B2/RConn1
  Hydraulic/LConn5 -- BPA2/RConn1
  Hydraulic/LConn6 -- B3/RConn1
  Hydraulic/LConn7 -- BPA3/RConn1
  Hydraulic/RConn1 -- N/RConn1

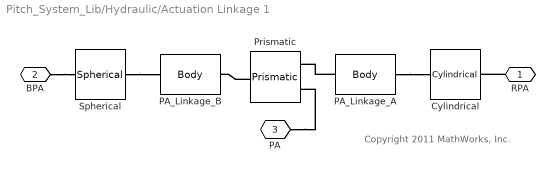
== system Pitch_System_Lib/Hydraulic/Actuation Linkage 1 ==
  note: Copyright 2011 MathWorks, Inc.
  Cylindrical : mblibv1/Joints/Cylindrical  PhysicalDomain=mechanical  SubClassName=Unknown  LeftPortType=blob  RightPortType=blob  LConnTagsString=__newl0  RConnTagsString=__newr0  UpdateFromCAD=off  NumSAPorts=0  CutJoint=off  MarkAsCut=off  Primitives=prismatic  PrimitiveProps=P1$Follower$[0 1 0]$prismatic#R1$Follower$[0 1 0]$revolute  DialogClass=JointBlock  P1Axis=[0 1 0]  R1Axis=[0 1 0]
  PA_Linkage_A : mblibv1/Bodies/Body  PhysicalDomain=mechanical  SubClassName=Unknown  LeftPortType=workingframe  RightPortType=workingframe  LConnTagsString=CS2  RConnTagsString=CS1  UpdateFromCAD=off  DialogClass=MechanicalBodyBlock  Mass=WT_Params.Pitch_Actuator.cylinder_mass  MassUnits=kg  InertiaUnits=kg*m^2  Inertia=WT_Params.Pitch_Actuator.cylinder_inertia  Shape=Cylinder  ShapeDims=[1 1]  ShapeUnits=m  ShapeUse=false  Density=1  DensityUnits=kg/m^3  DensityUse=false  GraphicsMode=MACHINE_DEFAULT  BodyColorSelMode=COLORPALETTE  BodyColor="[1     0.56863    0.011765]"  AttachedToCS=CG  CG=Left$CG$[WT_Params.Pitch_Actuator.cylinder_length/2 0 0]$CS2$CS2$m$[0 0 0]$Euler X-Y-Z$deg$CS1$false$none  WorkingFrames="Right$CS1$[WT_Params.Pitch_Actuator.cylinder_length 0 0]$CS2$CS2$m$[0 0 0]$Euler X-Y-Z$deg$Adjoining$true$none#Left$CS2$[0 0 0]$Adjoining$Adjoining$m$[0 0 0]$Euler X-Y-Z$deg$CS1$true$none#Right$CS7$[0 WT_Params.Pitch_Actuator.Geometry.outer_radius*cos(0)  WT_Params.Pitch_Actuator.Geometry.outer_radius*sin(0)]$CS1$CS1$m$[0 0 0]$Euler X-Y-Z$deg$CS1$false$none#Right$CS8$[0 WT_Params.Pitch_Actuator.Geometry.outer_radius*cos(0.2*pi)  WT_Params.Pitch_Actuator.Geometry.outer_radius*sin(0.2*pi)]$CS1$CS1$m$[0 0 0]$Euler X-Y-Z$deg$CS1$false$none#Right$CS9$[0 WT_Params.Pitch_Actuator.Geometry.outer_radius*cos(0.4*pi)  WT_Params.Pitch_Actuator.Geometry.outer_radius*sin(0.4*pi)]$CS1$CS1$m$[0 0 0]$Euler X-Y-Z$deg$CS1$false$none#Right$CS10$[0 WT_Params.Pitch_Actuator.Geometry.outer_radius*cos(0.6*pi)  WT_Params.Pitch_Actuator.Geometry.outer_radius*sin(0.6*pi)]$CS1$CS1$m$[0 0 0]$Euler X-Y-Z$deg$CS1$false$none#Right$CS11$[0 WT_Params.Pitch_Actuator.Geometry.outer_radius*cos(0.8*pi)  WT_Params.Pitch_Actuator.Geometry.outer_radius*sin(0.8*pi)]$CS1$CS1$m$[0 0 0]$Euler X-Y-Z$deg$CS1$false$none#Right$CS12$[0 WT_Params.Pitch_Actuator.Geometry.outer_radius*cos(1.0*pi)  WT_Params.Pitch_Actuator.Geometry.outer_radius*sin(1.0*pi)]$CS1$CS1$m$[0 0 0]$Euler X-Y-Z$deg$CS1$false$none#Right$CS13$[0 WT_Params.Pitch_Actuator.Geometry.outer_radius*cos(1.2*pi)  WT_Params.Pitch_Actuator.Geometry.outer_radius*sin(1.2*pi)]$CS1$CS1$m$[0 0 0]$Euler X-Y-Z$deg$CS1$false$none#Right$CS14$[0 WT_Params.Pitch_Actuator.Geometry.outer_radius*cos(1.4*pi)  WT_Params.Pitch_Actuator.Geometry.outer_radius*sin(1.4*pi)]$CS1$CS1$m$[0 0 0]$Euler X-Y-Z$deg$CS1$false$none#Right$CS15$[0 WT_Params.Pitch_Actuator.Geometry.outer_radius*cos(1.6*pi)  WT_Params.Pitch_Actuator.Geometry.outer_radius*sin(1.6*pi)]$CS1$CS1$m$[0 0 0]$Euler X-Y-Z$deg$CS1$false$none#Right$CS16$[0 WT_Params.Pitch_Actuator.Geometry.outer_radius*cos(1.8*pi)  WT_Params.Pitch_Actuator.Geometry.outer_radius*sin(1.8*pi)]$CS1$CS1$m$[0 0 0]$Euler X-Y-Z$deg$CS1$false$none#Right$CS17$[-WT_Params.Pitch_Actuator.cylinder_length WT_Params.Pitch_Actuator.Geometry.outer_radius*cos(0)  WT_Params.Pitch_Actuator.Geometry.outer_radius*sin(0)]$CS1$CS1$m$[0 0 0]$Euler X-Y-Z$deg$CS1$false$none#Right$CS18$[-WT_Params.Pitch_Actuator.cylinder_length WT_Params.Pitch_Actuator.Geometry.outer_radius*cos(0.2*pi)  WT_Params.Pitch_Actuator.Geometry.outer_radius*sin(0.2*pi)]$CS1$CS1$m$[0 0 0]$Euler X-Y-Z$deg$CS1$false$none#Right$CS19$[-WT_Params.Pitch_Actuator.cylinder_length WT_Params.Pitch_Actuator.Geometry.outer_radius*cos(0.4*pi)  WT_Params.Pitch_Actuator.Geometry.outer_radius*sin(0.4*pi)]$CS1$CS1$m$[0 0 0]$Euler X-Y-Z$deg$CS1$false$none#Right$CS20$[-WT_Params.Pitch_Actuator.cylinder_length WT_Params.Pitch_Actuator.Geometry.outer_radius*cos(0.6*pi)  WT_Params.Pitch_Actuator.Geometry.outer_radius*sin(0.6*pi)]$CS1$CS1$m$[0 0 0]$Euler X-Y-Z$deg$CS1$false$none#Right$CS21$[-WT_Params.Pitch_Actuator.cylinder_length WT_Params.Pitch_Actuator.Geometry.outer_radius*cos(0.8*pi)  WT_Params.Pitch_Actuator.Geometry.outer_radius*sin(0.8*pi)]$CS1$CS1$m$[0 0 0]$Euler X-Y-Z$deg$CS1$false$none#Right$CS22$[-WT_Params.Pitch_Actuator.cylinder_length WT_Params.Pitch_Actuator.Geometry.outer_radius*cos(1.0*pi)  WT_Params.Pitch_Actuator.Geometry.outer_radius*sin(1.0*pi)]$CS1$CS1$m$[0 0 0]$Euler X-Y-Z$deg$CS1$false$none#Right$CS23$[-WT_Params.Pitch_Actuator.cylinder_length WT_Params.Pitch_Actuator.Geometry.outer_radius*cos(1.2*pi)  WT_Params.Pitch_Actuator.Geometry.outer_radius*sin(1.2*pi)]$CS1$CS1$m$[0 0 0]$Euler X-Y-Z$deg$CS1$false$none#Right$CS24$[-WT_Params.Pitch_Actuator.cylinder_length WT_Params.Pitch_Actuator.Geometry.outer_radius*cos(1.4*pi)  WT_Params.Pitch_Actuator.Geometry.outer_radius*sin(1.4*pi)]$CS1$CS1$m$[0 0 0]$Euler X-Y-Z$deg$CS1$false$none#Right$CS25$[-WT_Params.Pitch_Actuator.cylinder_length WT_Params.Pitch_Actuator.Geometry.outer_radius*cos(1.6*pi)  WT_Params.Pitch_Actuator.Geometry.outer_radius*sin(1.6*pi)]$CS1$CS1$m$[0 0 0]$Euler X-Y-Z$deg$CS1$false$none#Right$CS26$[-WT_Params.Pitch_Actuator.cylinder_length WT_Params.Pitch_Actuator.Geometry.outer_radius*cos(1.8*pi)  WT_Params.Pitch_Actuator.Geometry.outer_radius*sin(1.8*pi)]$CS1$CS1$m$[0 0 0]$Euler X-Y-Z$deg$CS1$false$none"  CGPos=[WT_Params.Pitch_Actuator.cylinder_length/2 0 0]  CGRot=[0 0 0]  CS0Pos=[]  CS0Rot=[]  CS1Pos=[WT_Params.Pitch_Actuator.cylinder_length 0 0]  CS1Rot=[0 0 0]  CS2Pos=[0 0 0]  CS2Rot=[0 0 0]  CS3Pos=[]  CS3Rot=[]  CS4Pos=[]  CS4Rot=[]  CS5Pos=[]  CS5Rot=[]  CS6Pos=[]  CS6Rot=[]  CS7Pos="[0 WT_Params.Pitch_Actuator.Geometry.outer_radius*cos(0)  WT_Params.Pitch_Actuator.Geometry.outer_radius*sin(0)]"  CS7Rot=[0 0 0]  CS8Pos="[0 WT_Params.Pitch_Actuator.Geometry.outer_radius*cos(0.2*pi)  WT_Params.Pitch_Actuator.Geometry.outer_radius*sin(0.2*pi)]"  CS8Rot=[0 0 0]  CS9Pos="[0 WT_Params.Pitch_Actuator.Geometry.outer_radius*cos(0.4*pi)  WT_Params.Pitch_Actuator.Geometry.outer_radius*sin(0.4*pi)]"  CS9Rot=[0 0 0]  CS10Pos="[0 WT_Params.Pitch_Actuator.Geometry.outer_radius*cos(0.6*pi)  WT_Params.Pitch_Actuator.Geometry.outer_radius*sin(0.6*pi)]"  CS10Rot=[0 0 0]  CS11Pos="[0 WT_Params.Pitch_Actuator.Geometry.outer_radius*cos(0.8*pi)  WT_Params.Pitch_Actuator.Geometry.outer_radius*sin(0.8*pi)]"  CS11Rot=[0 0 0]  CS12Pos="[0 WT_Params.Pitch_Actuator.Geometry.outer_radius*cos(1.0*pi)  WT_Params.Pitch_Actuator.Geometry.outer_radius*sin(1.0*pi)]"  CS12Rot=[0 0 0]  CS13Pos="[0 WT_Params.Pitch_Actuator.Geometry.outer_radius*cos(1.2*pi)  WT_Params.Pitch_Actuator.Geometry.outer_radius*sin(1.2*pi)]"  CS13Rot=[0 0 0]  CS14Pos="[0 WT_Params.Pitch_Actuator.Geometry.outer_radius*cos(1.4*pi)  WT_Params.Pitch_Actuator.Geometry.outer_radius*sin(1.4*pi)]"  CS14Rot=[0 0 0]  CS15Pos="[0 WT_Params.Pitch_Actuator.Geometry.outer_radius*cos(1.6*pi)  WT_Params.Pitch_Actuator.Geometry.outer_radius*sin(1.6*pi)]"  CS15Rot=[0 0 0]  CS16Pos="[0 WT_Params.Pitch_Actuator.Geometry.outer_radius*cos(1.8*pi)  WT_Params.Pitch_Actuator.Geometry.outer_radius*sin(1.8*pi)]"  CS16Rot=[0 0 0]  CS17Pos="[-WT_Params.Pitch_Actuator.cylinder_length WT_Params.Pitch_Actuator.Geometry.outer_radius*cos(0)  WT_Params.Pitch_Actuator.Geometry.outer_radius*sin(0)]"  CS17Rot=[0 0 0]  CS18Pos="[-WT_Params.Pitch_Actuator.cylinder_length WT_Params.Pitch_Actuator.Geometry.outer_radius*cos(0.2*pi)  WT_Params.Pitch_Actuator.Geometry.outer_radius*sin(0.2*pi)]"  CS18Rot=[0 0 0]  CS19Pos="[-WT_Params.Pitch_Actuator.cylinder_length WT_Params.Pitch_Actuator.Geometry.outer_radius*cos(0.4*pi)  WT_Params.Pitch_Actuator.Geometry.outer_radius*sin(0.4*pi)]"  CS19Rot=[0 0 0]  CS20Pos="[-WT_Params.Pitch_Actuator.cylinder_length WT_Params.Pitch_Actuator.Geometry.outer_radius*cos(0.6*pi)  WT_Params.Pitch_Actuator.Geometry.outer_radius*sin(0.6*pi)]"  CS20Rot=[0 0 0]
  PA_Linkage_B : mblibv1/Bodies/Body  PhysicalDomain=mechanical  SubClassName=Unknown  LeftPortType=workingframe  RightPortType=workingframe  LConnTagsString=CS2  RConnTagsString=CS1  UpdateFromCAD=off  DialogClass=MechanicalBodyBlock  Mass=WT_Params.Pitch_Actuator.rod_mass  MassUnits=kg  InertiaUnits=kg*m^2  Inertia=WT_Params.Pitch_Actuator.rod_inertia  Shape=Cylinder  ShapeDims=[1 1]  ShapeUnits=m  ShapeUse=false  Density=1  DensityUnits=kg/m^3  DensityUse=false  GraphicsMode=MACHINE_DEFAULT  BodyColorSelMode=COLORPALETTE  BodyColor="[0.31373     0.31765     0.31373]"  AttachedToCS=CG  CG=Left$CG$[-WT_Params.Pitch_Actuator.cylinder_length/2 0 0]$CS1$CS1$m$[0 0 0]$Euler X-Y-Z$deg$CS1$false$none  WorkingFrames="Right$CS1$[0 0 0]$Adjoining$Adjoining$m$[0 0 0]$Euler X-Y-Z$deg$Adjoining$true$none#Left$CS2$[-WT_Params.Pitch_Actuator.cylinder_length 0 0]$CS1$CS1$m$[0 0 0]$Euler X-Y-Z$deg$CS1$true$none#Right$CS7$[0 WT_Params.Pitch_Actuator.Geometry.inner_radius*cos(0)  WT_Params.Pitch_Actuator.Geometry.inner_radius*sin(0)]$CS1$CS1$m$[0 0 0]$Euler X-Y-Z$deg$CS1$false$none#Right$CS8$[0 WT_Params.Pitch_Actuator.Geometry.inner_radius*cos(0.2*pi)  WT_Params.Pitch_Actuator.Geometry.inner_radius*sin(0.2*pi)]$CS1$CS1$m$[0 0 0]$Euler X-Y-Z$deg$CS1$false$none#Right$CS9$[0 WT_Params.Pitch_Actuator.Geometry.inner_radius*cos(0.4*pi)  WT_Params.Pitch_Actuator.Geometry.inner_radius*sin(0.4*pi)]$CS1$CS1$m$[0 0 0]$Euler X-Y-Z$deg$CS1$false$none#Right$CS10$[0 WT_Params.Pitch_Actuator.Geometry.inner_radius*cos(0.6*pi)  WT_Params.Pitch_Actuator.Geometry.inner_radius*sin(0.6*pi)]$CS1$CS1$m$[0 0 0]$Euler X-Y-Z$deg$CS1$false$none#Right$CS11$[0 WT_Params.Pitch_Actuator.Geometry.inner_radius*cos(0.8*pi)  WT_Params.Pitch_Actuator.Geometry.inner_radius*sin(0.8*pi)]$CS1$CS1$m$[0 0 0]$Euler X-Y-Z$deg$CS1$false$none#Right$CS12$[0 WT_Params.Pitch_Actuator.Geometry.inner_radius*cos(1.0*pi)  WT_Params.Pitch_Actuator.Geometry.inner_radius*sin(1.0*pi)]$CS1$CS1$m$[0 0 0]$Euler X-Y-Z$deg$CS1$false$none#Right$CS13$[0 WT_Params.Pitch_Actuator.Geometry.inner_radius*cos(1.2*pi)  WT_Params.Pitch_Actuator.Geometry.inner_radius*sin(1.2*pi)]$CS1$CS1$m$[0 0 0]$Euler X-Y-Z$deg$CS1$false$none#Right$CS14$[0 WT_Params.Pitch_Actuator.Geometry.inner_radius*cos(1.4*pi)  WT_Params.Pitch_Actuator.Geometry.inner_radius*sin(1.4*pi)]$CS1$CS1$m$[0 0 0]$Euler X-Y-Z$deg$CS1$false$none#Right$CS15$[0 WT_Params.Pitch_Actuator.Geometry.inner_radius*cos(1.6*pi)  WT_Params.Pitch_Actuator.Geometry.inner_radius*sin(1.6*pi)]$CS1$CS1$m$[0 0 0]$Euler X-Y-Z$deg$CS1$false$none#Right$CS16$[0 WT_Params.Pitch_Actuator.Geometry.inner_radius*cos(1.8*pi)  WT_Params.Pitch_Actuator.Geometry.inner_radius*sin(1.8*pi)]$CS1$CS1$m$[0 0 0]$Euler X-Y-Z$deg$CS1$false$none#Right$CS17$[-WT_Params.Pitch_Actuator.cylinder_length WT_Params.Pitch_Actuator.Geometry.inner_radius*cos(0)  WT_Params.Pitch_Actuator.Geometry.inner_radius*sin(0)]$CS1$CS1$m$[0 0 0]$Euler X-Y-Z$deg$CS1$false$none#Right$CS18$[-WT_Params.Pitch_Actuator.cylinder_length WT_Params.Pitch_Actuator.Geometry.inner_radius*cos(0.2*pi)  WT_Params.Pitch_Actuator.Geometry.inner_radius*sin(0.2*pi)]$CS1$CS1$m$[0 0 0]$Euler X-Y-Z$deg$CS1$false$none#Right$CS19$[-WT_Params.Pitch_Actuator.cylinder_length WT_Params.Pitch_Actuator.Geometry.inner_radius*cos(0.4*pi)  WT_Params.Pitch_Actuator.Geometry.inner_radius*sin(0.4*pi)]$CS1$CS1$m$[0 0 0]$Euler X-Y-Z$deg$CS1$false$none#Right$CS20$[-WT_Params.Pitch_Actuator.cylinder_length WT_Params.Pitch_Actuator.Geometry.inner_radius*cos(0.6*pi)  WT_Params.Pitch_Actuator.Geometry.inner_radius*sin(0.6*pi)]$CS1$CS1$m$[0 0 0]$Euler X-Y-Z$deg$CS1$false$none#Right$CS21$[-WT_Params.Pitch_Actuator.cylinder_length WT_Params.Pitch_Actuator.Geometry.inner_radius*cos(0.8*pi)  WT_Params.Pitch_Actuator.Geometry.inner_radius*sin(0.8*pi)]$CS1$CS1$m$[0 0 0]$Euler X-Y-Z$deg$CS1$false$none#Right$CS22$[-WT_Params.Pitch_Actuator.cylinder_length WT_Params.Pitch_Actuator.Geometry.inner_radius*cos(1.0*pi)  WT_Params.Pitch_Actuator.Geometry.inner_radius*sin(1.0*pi)]$CS1$CS1$m$[0 0 0]$Euler X-Y-Z$deg$CS1$false$none#Right$CS23$[-WT_Params.Pitch_Actuator.cylinder_length WT_Params.Pitch_Actuator.Geometry.inner_radius*cos(1.2*pi)  WT_Params.Pitch_Actuator.Geometry.inner_radius*sin(1.2*pi)]$CS1$CS1$m$[0 0 0]$Euler X-Y-Z$deg$CS1$false$none#Right$CS24$[-WT_Params.Pitch_Actuator.cylinder_length WT_Params.Pitch_Actuator.Geometry.inner_radius*cos(1.4*pi)  WT_Params.Pitch_Actuator.Geometry.inner_radius*sin(1.4*pi)]$CS1$CS1$m$[0 0 0]$Euler X-Y-Z$deg$CS1$false$none#Right$CS25$[-WT_Params.Pitch_Actuator.cylinder_length WT_Params.Pitch_Actuator.Geometry.inner_radius*cos(1.6*pi)  WT_Params.Pitch_Actuator.Geometry.inner_radius*sin(1.6*pi)]$CS1$CS1$m$[0 0 0]$Euler X-Y-Z$deg$CS1$false$none#Right$CS26$[-WT_Params.Pitch_Actuator.cylinder_length WT_Params.Pitch_Actuator.Geometry.inner_radius*cos(1.8*pi)  WT_Params.Pitch_Actuator.Geometry.inner_radius*sin(1.8*pi)]$CS1$CS1$m$[0 0 0]$Euler X-Y-Z$deg$CS1$false$none"  CGPos=[-WT_Params.Pitch_Actuator.cylinder_length/2 0 0]  CGRot=[0 0 0]  CS0Pos=[]  CS0Rot=[]  CS1Pos=[0 0 0]  CS1Rot=[0 0 0]  CS2Pos=[-WT_Params.Pitch_Actuator.cylinder_length 0 0]  CS2Rot=[0 0 0]  CS3Pos=[]  CS3Rot=[]  CS4Pos=[]  CS4Rot=[]  CS5Pos=[]  CS5Rot=[]  CS6Pos=[]  CS6Rot=[]  CS7Pos="[0 WT_Params.Pitch_Actuator.Geometry.inner_radius*cos(0)  WT_Params.Pitch_Actuator.Geometry.inner_radius*sin(0)]"  CS7Rot=[0 0 0]  CS8Pos="[0 WT_Params.Pitch_Actuator.Geometry.inner_radius*cos(0.2*pi)  WT_Params.Pitch_Actuator.Geometry.inner_radius*sin(0.2*pi)]"  CS8Rot=[0 0 0]  CS9Pos="[0 WT_Params.Pitch_Actuator.Geometry.inner_radius*cos(0.4*pi)  WT_Params.Pitch_Actuator.Geometry.inner_radius*sin(0.4*pi)]"  CS9Rot=[0 0 0]  CS10Pos="[0 WT_Params.Pitch_Actuator.Geometry.inner_radius*cos(0.6*pi)  WT_Params.Pitch_Actuator.Geometry.inner_radius*sin(0.6*pi)]"  CS10Rot=[0 0 0]  CS11Pos="[0 WT_Params.Pitch_Actuator.Geometry.inner_radius*cos(0.8*pi)  WT_Params.Pitch_Actuator.Geometry.inner_radius*sin(0.8*pi)]"  CS11Rot=[0 0 0]  CS12Pos="[0 WT_Params.Pitch_Actuator.Geometry.inner_radius*cos(1.0*pi)  WT_Params.Pitch_Actuator.Geometry.inner_radius*sin(1.0*pi)]"  CS12Rot=[0 0 0]  CS13Pos="[0 WT_Params.Pitch_Actuator.Geometry.inner_radius*cos(1.2*pi)  WT_Params.Pitch_Actuator.Geometry.inner_radius*sin(1.2*pi)]"  CS13Rot=[0 0 0]  CS14Pos="[0 WT_Params.Pitch_Actuator.Geometry.inner_radius*cos(1.4*pi)  WT_Params.Pitch_Actuator.Geometry.inner_radius*sin(1.4*pi)]"  CS14Rot=[0 0 0]  CS15Pos="[0 WT_Params.Pitch_Actuator.Geometry.inner_radius*cos(1.6*pi)  WT_Params.Pitch_Actuator.Geometry.inner_radius*sin(1.6*pi)]"  CS15Rot=[0 0 0]  CS16Pos="[0 WT_Params.Pitch_Actuator.Geometry.inner_radius*cos(1.8*pi)  WT_Params.Pitch_Actuator.Geometry.inner_radius*sin(1.8*pi)]"  CS16Rot=[0 0 0]  CS17Pos="[-WT_Params.Pitch_Actuator.cylinder_length WT_Params.Pitch_Actuator.Geometry.inner_radius*cos(0)  WT_Params.Pitch_Actuator.Geometry.inner_radius*sin(0)]"  CS17Rot=[0 0 0]  CS18Pos="[-WT_Params.Pitch_Actuator.cylinder_length WT_Params.Pitch_Actuator.Geometry.inner_radius*cos(0.2*pi)  WT_Params.Pitch_Actuator.Geometry.inner_radius*sin(0.2*pi)]"  CS18Rot=[0 0 0]  CS19Pos="[-WT_Params.Pitch_Actuator.cylinder_length WT_Params.Pitch_Actuator.Geometry.inner_radius*cos(0.4*pi)  WT_Params.Pitch_Actuator.Geometry.inner_radius*sin(0.4*pi)]"  CS19Rot=[0 0 0]  CS20Pos="[-WT_Params.Pitch_Actuator.cylinder_length WT_Params.Pitch_Actuator.Geometry.inner_radius*cos(0.6*pi)  WT_Params.Pitch_Actuator.Geometry.inner_radius*sin(0.6*pi)]"  CS20Rot=[0 0 0]
  Prismatic : mblibv1/Joints/Prismatic  PhysicalDomain=mechanical  SubClassName=Unknown  LeftPortType=blob  RightPortType=blob  LConnTagsString=__newl0|SA1  RConnTagsString=__newr0  UpdateFromCAD=off  NumSAPorts=1  CutJoint=off  MarkAsCut=off  Primitives=prismatic  PrimitiveProps=P1$Base$[1 0 0]$prismatic  DialogClass=JointBlock  P1Axis=[1 0 0]
  Spherical : mblibv1/Joints/Spherical  LConnTagsString=__newl0  RConnTagsString=__newr0  UpdateFromCAD=off  NumSAPorts=0  CutJoint=off  MarkAsCut=off  Primitives=spherical  PrimitiveProps=S$WORLD$[0 0 0]$spherical  DialogClass=JointBlock  SAxis=[0 0 0]
  RPA : PMIOPort  Port=1  Side=Right
  BPA : PMIOPort  Port=2  Side=Left
  PA : PMIOPort  Tag=PMCPort  Port=3  Side=Left
  connections:
  BPA/RConn1 -- Spherical/LConn1
  RPA/RConn1 -- Cylindrical/RConn1
  PA/RConn1 -- Prismatic/LConn2
  Prismatic/RConn1 -- PA_Linkage_B/LConn1
  Spherical/RConn1 -- PA_Linkage_B/RConn1
  PA_Linkage_A/LConn1 -- Cylindrical/LConn1
  PA_Linkage_A/RConn1 -- Prismatic/LConn1
